simulink model "virtuallab2"  (R2017b)
settings: Solver=VariableStepAuto  StartTime=0.0  StopTime=10.0  RelTol=1e-3
settings Model: Creator=Nick  LastModifiedBy=Nick

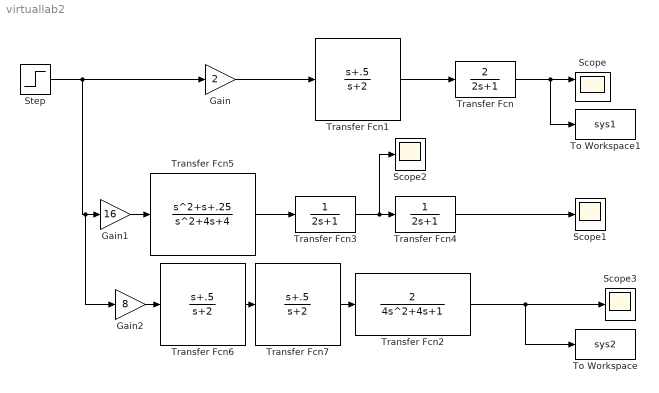
== system virtuallab2 ==
  Gain : Gain  Gain=2
  Gain1 : Gain  Gain=16
  Gain2 : Gain  Gain=8
  Scope : Scope  NumInputPorts=2
  Scope1 : Scope
  Scope2 : Scope
  Scope3 : Scope
  Step : Step  Time=0  SampleTime=0
  To Workspace : ToWorkspace  VariableName=sys2  SaveFormat=Timeseries  SampleTime=-1
  To Workspace1 : ToWorkspace  VariableName=sys1  SaveFormat=Timeseries  SampleTime=-1
  Transfer Fcn : TransferFcn  Numerator=[2]  Denominator=[2 1]
  Transfer Fcn1 : TransferFcn  Numerator=[1 .5]  Denominator=[ 1 2]
  Transfer Fcn2 : TransferFcn  Numerator=[2]  Denominator=[4 4 1]
  Transfer Fcn3 : TransferFcn  Denominator=[2 1]
  Transfer Fcn4 : TransferFcn  Denominator=[2 1]
  Transfer Fcn5 : TransferFcn  Numerator=[1 1 .25]  Denominator=[ 1 4 4]
  Transfer Fcn6 : TransferFcn  Numerator=[1 .5]  Denominator=[ 1 2]
  Transfer Fcn7 : TransferFcn  Numerator=[1 .5]  Denominator=[ 1 2]
  wires:
  Transfer Fcn/1 -> To Workspace1/1, Scope/1
  Transfer Fcn1/1 -> Transfer Fcn/1
  Gain/1 -> Transfer Fcn1/1
  Transfer Fcn3/1 -> Transfer Fcn4/1, Scope2/1
  Transfer Fcn4/1 -> Scope1/1
  Transfer Fcn5/1 -> Transfer Fcn3/1
  Gain1/1 -> Transfer Fcn5/1
  Step/1 -> Gain2/1, Gain1/1, Gain/1
  Transfer Fcn7/1 -> Transfer Fcn2/1
  Gain2/1 -> Transfer Fcn6/1
  Transfer Fcn2/1 -> Scope3/1, To Workspace/1
  Transfer Fcn6/1 -> Transfer Fcn7/1
